simulink model "experimentHarness"  (R2025b)
settings: Solver=VariableStepAuto  StartTime=0.0  StopTime=10.0  RelTol=1e-3
undefined symbols (not defined in the file): scenario
settings Model: Creator=jaiden  LastModifiedBy=jaiden

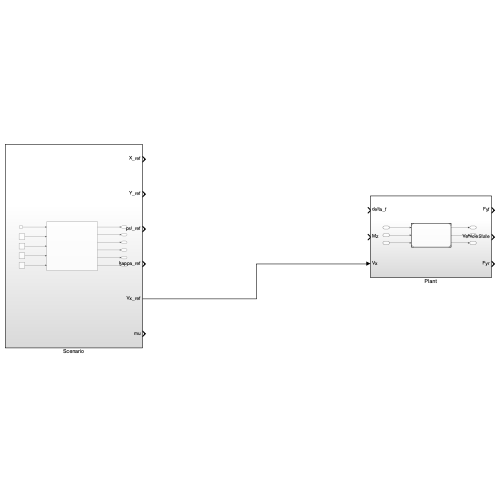
[thumbnail: Simulink's stored preview of the top-level diagram]
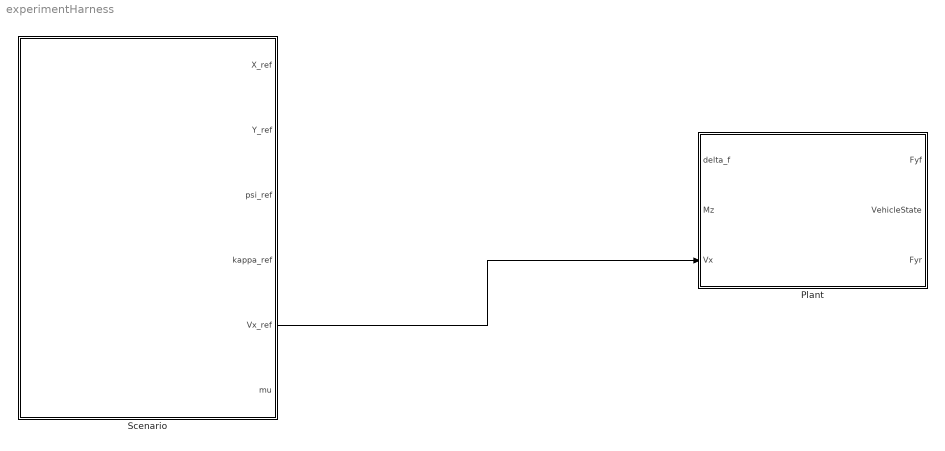
== system experimentHarness ==
  Plant : Subsystem
  Scenario : Subsystem
  wires:
  Scenario/5(Vx_ref) -> Plant/3(Vx)

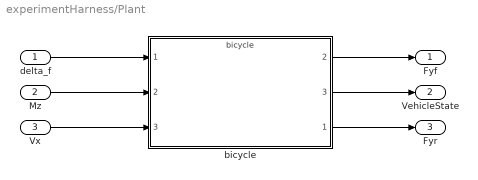
== system experimentHarness/Plant ==
  delta_f : Inport
  Mz : Inport  Port=2
  Vx : Inport  Port=3
  bicycle : ModelReference  ModelNameDialog=bicycle.slx  SimulationMode=Normal  ModelReferenceVersion=1.4
      settings: PortSchema="{\"entries\":[{\"content\":{\"sides\":[{\"content\":{\"connectorIds\":[\"In1\",\"In2\",\"In3\"]},\"type\":\"ConnectorPlacement.EquallySpacedRectSide\",\"uuid\":\"58d1b5ba-aa94-409a-86bc-1f2a380b806f\"},{\"content\":{\"connectorIds\":[\"Out2\",\"Out3\",\"Out1\"],\"side\":\"RIGHT\"},\"type\":\"ConnectorPlacement.EquallySpacedRectSide\",\"uuid\":\"d4837c49-e6bf-462c-b169-66ee2b0f1817\"},{\"content\":{\"side\":\"TOP\"},\"type\":\"ConnectorPlacement.EquallySpacedRectSide\",\"uuid\":\"4cad5275-f3ab-4015-917f-efe21967d551\"}]},\"type\":\"ConnectorPlacement.EquallySpacedConnector\",\"uuid\":\"b91e3d72-bb0a-4328-b099-f36bf503b2b7\"}],\"packageUris\":[\"http://schema.mathworks.com/mf0/Connector/R2020b\"],\"version\":\"1.0\"}"
  Fyf : Outport
  VehicleState : Outport  Port=2
  Fyr : Outport  Port=3
  wires:
  delta_f/1 -> bicycle/1
  Mz/1 -> bicycle/2
  Vx/1 -> bicycle/3
  bicycle/3 -> VehicleState/1
  bicycle/2 -> Fyf/1
  bicycle/1 -> Fyr/1

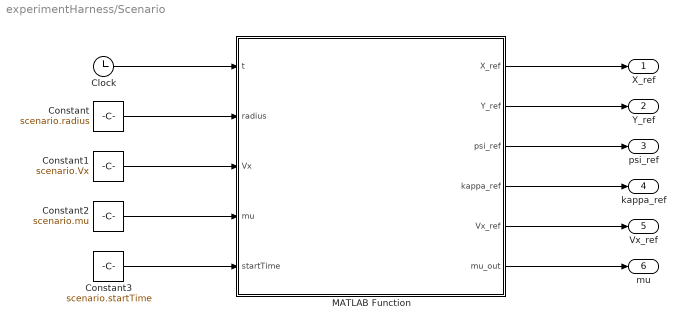
== system experimentHarness/Scenario ==
  Clock : Clock
  Constant : Constant  Value=scenario.radius
  Constant1 : Constant  Value=scenario.Vx
  Constant2 : Constant  Value=scenario.mu
  Constant3 : Constant  Value=scenario.startTime
  MATLAB Function : MATLAB Function  TreatAsAtomicUnit=on
  X_ref : Outport
  Y_ref : Outport  Port=2
  psi_ref : Outport  Port=3
  kappa_ref : Outport  Port=4
  Vx_ref : Outport  Port=5
  mu : Outport  Port=6
  wires:
  Clock/1 -> MATLAB Function/1(t)
  Constant/1 -> MATLAB Function/2(radius)
  Constant1/1 -> MATLAB Function/3(Vx)
  Constant2/1 -> MATLAB Function/4(mu)
  Constant3/1 -> MATLAB Function/5(startTime)
  MATLAB Function/1(X_ref) -> X_ref/1
  MATLAB Function/2(Y_ref) -> Y_ref/1
  MATLAB Function/3(psi_ref) -> psi_ref/1
  MATLAB Function/4(kappa_ref) -> kappa_ref/1
  MATLAB Function/5(Vx_ref) -> Vx_ref/1
  MATLAB Function/6(mu_out) -> mu/1

== matlab function experimentHarness/Scenario/MATLAB Function ==
  data: t input; X_ref output; radius input; Vx input; mu input; startTime input; Y_ref output; psi_ref output; kappa_ref output; Vx_ref output; mu_out output
function [X_ref, Y_ref, psi_ref, kappa_ref, Vx_ref, mu_out] = ...
    curvedLaneReference(t, radius, Vx, mu, startTime)

Vx_ref = Vx;
mu_out = mu;

if t < startTime
    % Initial straight section
    X_ref = Vx*t;
    Y_ref = 0;
    psi_ref = 0;
    kappa_ref = 0;
else
    % Constant-radius curved section
    X0 = Vx*startTime;
    theta = Vx*(t - startTime)/radius;

    X_ref = X0 + radius*sin(theta);
    Y_ref = radius*(1 - cos(theta));
    psi_ref = theta;
    kappa_ref = 1/radius;
end

end
